simulink model "Roll_Diff_SS_C"  (R2013a)
settings: Solver=ode45  StartTime=0.0  StopTime=sim_length  RelTol=1e-3
values from neighbouring files (symbols this model uses):
  K_Roll_C = place(A,B,[p1 p2 p3])    [State_Space_Roll_C.m]
  Nbar_Roll_C = Nbar(1)    [State_Space_Roll_C.m]
undefined symbols (not defined in the file or in its folder): I_Theta, Kf, L, Motor_TimeConstant
settings Model: Creator=Ross  LastModifiedBy=Ross

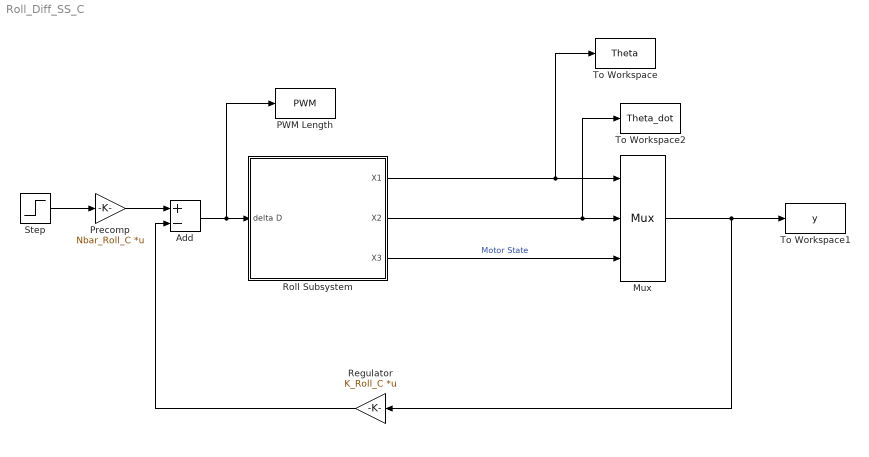
== system Roll_Diff_SS_C ==
  Add : Sum  Inputs=+-
  Mux : Mux  Inputs=3
      settings: DisplayOption=signals
  PWM Length : ToWorkspace  VariableName=PWM  SampleTime=-1  SaveFormat=Timeseries
  Precomp : Gain  Gain=Nbar_Roll_C  Multiplication=Matrix(K*u)
  Regulator : Gain  Gain=K_Roll_C  Multiplication=Matrix(K*u)
  Roll Subsystem : Subsystem
  Step : Step  SampleTime=0
  To Workspace : ToWorkspace  VariableName=Theta  SampleTime=-1  SaveFormat=Timeseries
  To Workspace1 : ToWorkspace  VariableName=y  SampleTime=-1
  To Workspace2 : ToWorkspace  VariableName=Theta_dot  SampleTime=-1  SaveFormat=Timeseries
  wires:
  Roll Subsystem/1(X1) -> To Workspace/1, Mux/1
  Roll Subsystem/2(X2) -> To Workspace2/1, Mux/2
  Mux/1 -> Regulator/1, To Workspace1/1
  Roll Subsystem/3(X3) -> Mux/3  "Motor State"
  Add/1 -> PWM Length/1, Roll Subsystem/1(delta D)
  Step/1 -> Precomp/1
  Regulator/1 -> Add/2
  Precomp/1 -> Add/1

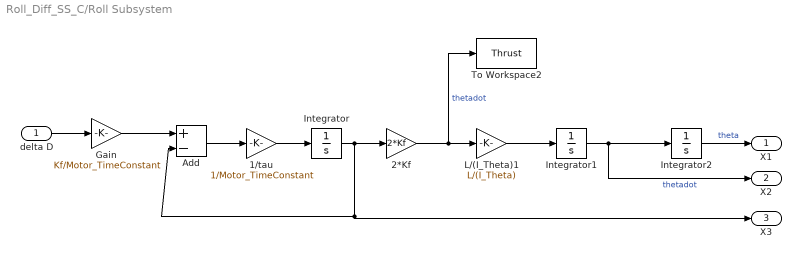
== system Roll_Diff_SS_C/Roll Subsystem ==
  delta D : Inport
  1/tau : Gain  Gain=1/Motor_TimeConstant
  2*Kf : Gain  Gain=2*Kf
  Add : Sum  Inputs=+-
  Gain : Gain  Gain=Kf/Motor_TimeConstant
  Integrator : Integrator
  Integrator1 : Integrator
  Integrator2 : Integrator
  L/(I_Theta)1 : Gain  Gain=L/(I_Theta)
  To Workspace2 : ToWorkspace  VariableName=Thrust  SampleTime=-1  SaveFormat=Timeseries
  X1 : Outport
  X2 : Outport  Port=2
  X3 : Outport  Port=3
  wires:
  2*Kf/1 -> To Workspace2/1, L/(I_Theta)1/1  "thetadot"
  Integrator2/1 -> X1/1  "theta"
  Add/1 -> 1/tau/1
  Gain/1 -> Add/1
  delta D/1 -> Gain/1
  Integrator/1 -> 2*Kf/1, Add/2, X3/1
  1/tau/1 -> Integrator/1
  Integrator1/1 -> Integrator2/1, X2/1  "thetadot"
  L/(I_Theta)1/1 -> Integrator1/1
